simulink model "HybridMicrogrid_FuzzyLogic"  (R2024b)
settings: Solver=ode23tb  StartTime=0.0  StopTime=86000  RelTol=1e-3
PreLoadFcn:
  | addpath('Resources')
InitFcn:
  | initialConditions();
libraries: simulink x6, spsThreePhaseDynamicLoadLib x4, spsThreePhaseVIMeasurementLib x4, spsPower3phPhasorLib x3, spsThreePhaseBreakerLib x3, spsThreePhaseSourceLib x2, fuzblock x2, spsFrequencyPhasorLib x2, spsSequenceAnalyzerPhasorLib x2, powerlib_meascontrol x1, powerlib x1, spsCurrentMeasurementLib x1
settings Model: SimulationMode=accelerator  Creator=jlesage  LastModifiedBy=RDBNTO016
settings SolverCC: ZeroCrossAlgorithm=Adaptive  AlgebraicLoopSolver=TrustRegion
settings DataIOCC: ReturnWorkspaceOutputs=off
settings DebuggingCC: IgnoredZcDiagnostic=none  PregeneratedLibrarySubsystemCodeDiagnostic=none  ArithmeticOperatorsInVariantConditions=warning
settings ModelReferenceCC: EnableRefExpFcnMdlSchedulingChecks=on
settings SFSimCC: SimUseLocalCustomCode=off  CustomCodeUndefinedFunction=UseInterfaceOnly
settings RTWCC: RTWUseLocalCustomCode=off  GPUComputeCapability=3.5

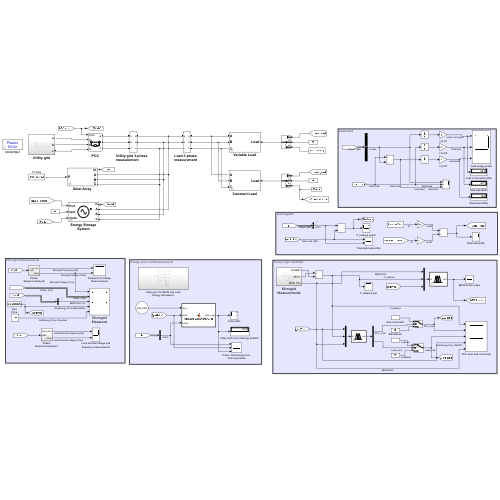
[thumbnail: Simulink's stored preview of the top-level diagram]
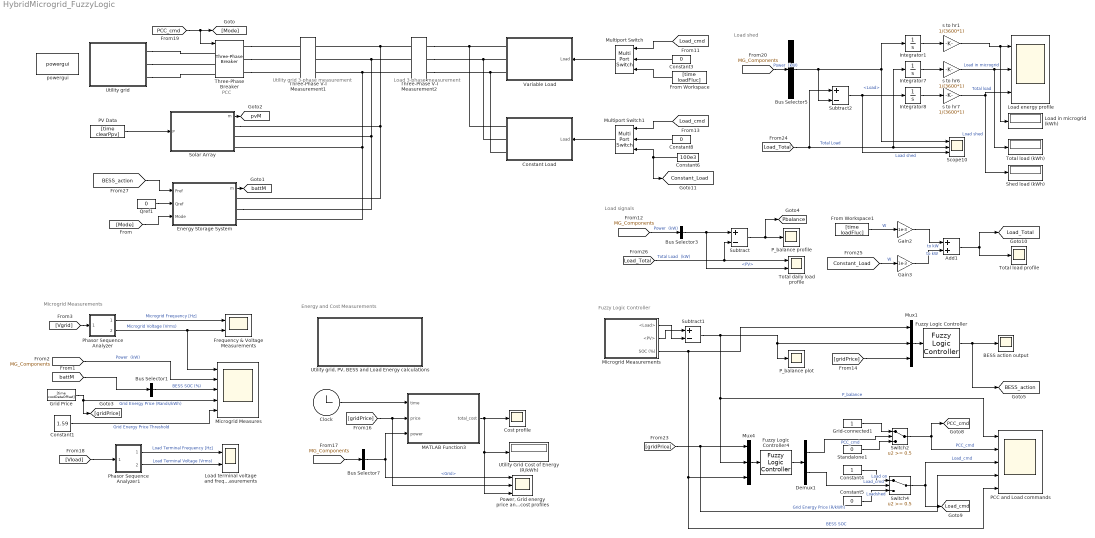
== system HybridMicrogrid_FuzzyLogic ==
  note: PCC
  note: Energy and Cost Measurements
  note: Fuzzy Logic Controller
  note: Microgrid Measurements
  note: Load shed
  note: Load 3-phase measurement
  note: Utility grid 3-phase measurement
  note: Load signals
  Add1 : Sum
  BESS action output : Scope
  Bus Selector1 : BusSelector  OutputSignals=SOC (%)  OutputAsBus=on
  Bus Selector3 : BusSelector  OutputSignals=PV
  Bus Selector5 : BusSelector  OutputSignals=Load
  Bus Selector7 : BusSelector  OutputSignals=Grid
  Clock : Clock
  Constant Load : Subsystem  mask(Variable Load (PQ Model)){Vn=400, Fn=50, PF=1, Load0=0}
      mask prompts: Vn "Nominal L-L Voltage [Vrms]"; Fn "Nominal Frequency [Hz]"; PF "Power Factor [0 to 1]"; Load0 "Initial Load [W]"
      mask help:
      | The Variable Load block is a lumped approximation for a distribution feeder. For non-unity power factor loads, the input (active power) is scaled accordingly to generate a desired load.
      |
      | Note: The initial input load must be specified for use for Load Flow analysis.
      mask init:
      | P0 = Load0;
      | Q0 = Load0*sqrt(1/PF^2-1);
      mask Display:
      | port_label('input',1,'Load')
      | port_label('Rconn',1,'A')
      | port_label('Rconn',2,'B')
      | port_label('Rconn',3,'C')
  Constant1 : Constant  Value=1.59
  Constant3 : Constant  Value=0
  Constant4 : Constant
  Constant5 : Constant  Value=0
  Constant6 : Constant  Value=100e3
  Constant8 : Constant  Value=0
  Cost profile : Scope
  Demux1 : Demux  Outputs=2
  Energy Storage System : Subsystem  mask(Grid-connected Energy Storage (PQ Model)){SimMode=Phasor, Vn=400, Fn=50, PnomkW=300, kWh_Rated=3000, Efficiency=96, LimitVec=[90 30], RechargeSOC=50, Precharge=90, autoRecharge=on, Initial_kWh_pc=50, PQvec=[300e3 0]}
      mask prompts: SimMode "Simulation Mode"; Vn "Nominal L-L Voltage [Vrms]"; Fn "Nominal Frequency [Hz]"; PnomkW "Rated Power [kW]"; kWh_Rated "Rated Capacity [kWh]"; Efficiency "Overall System Efficiency [%]"; LimitVec "Upper/Lower Charge Limits [%]"; RechargeSOC "SOC to Recharge [%]"; Precharge "Recharge Rate [% of Rated Power]"; autoRecharge "Enable Auto-Recharge"; Initial_kWh_pc "Initial State-of-Charge [0-100%]"; PQvec "Initial Active/Reactive Cmds"
      mask help:
      | The energy storage block models a generic grid-connected energy storage system (ESS), most commonly a battery system. This is a system-level model that does not contain any power electronics, but is useful for load flow, phasor, and hybrid phasor-EMT simulations. The inputs to this block are the commanded active and reactive power of the ESS. The ESS is assumed to have four quadrent operation. The Mode Input dictates what high-level operation the ESS has: current control (Mode = 1) or voltage control (Mode = 0). Current control is ideal for a grid connected system where you need to specify P,Q commands. Voltage control is necessary if the ESS will be the only system supporting the microgrid in islanded mode.
      |
      | For more detailed ESS models, consider the battery block in the Drives library. Consider using this PQ Model to perform load flow studies and switch to a more detailed model when full EMT studies or more advanced controls are required.
      |
      | Note: The initial active/reactive power commands must be specified for use for Load Flow analysis.
      mask init:
      | % Calculate Initial Conditions
      | Pnom = PnomkW*1e3;
      | P0 = -PQvec(1);  Q0 = -PQvec(2);
      | if abs(P0) > Pnom
      |     P0 = sign(P0)*Pnom;
      | end
      | 
      | % Calculate Q0 given Reactive Power Capability Curve
      | Qlim = sqrt(Pnom^2 - P0^2);
      | if Qlim > abs(Q0)
      |     Q0 = sign(Q0)*Qlim;
      | end
      | 
      | UpChrgLim = LimitVec(1);
      | LowChrgLim = LimitVec(2);
      | if Initial_kWh_pc > UpChrgLim && P0 < 0
      |     P0 = 0; Q0 = 0;
      | elseif Initial_kWh_pc < LowChrgLim && P0 > 0
      |     P0 = 0; Q0 = 0;
      | end
      | 
      | simulationStatus =  get_param(bdroot,'SimulationStatus');
      | 
      | % The active variant can only be modified at edit-time or very early during
      | % the simulink compile stage. 
      | if any(strcmp(simulationStatus, {'stopped'}))
      | 
      | blk = [gcb '/Power Measures'];
      | if strcmp(SimMode,'Phasor')
      |     set_param(blk,'OverrideUsingVariant','Phasor');
      | else
      |     set_param(blk,'OverrideUsingVariant','EMT');
      | end
      | 
      | 
      | end
      mask TypeOptions SimMode: Electromagnetic Transient (EMT) | Phasor
      mask DialogControl Container7 Prompt: Grid Connection Properties
      mask DialogControl Container11 Prompt: Charge/Discharge Controls
      mask DialogControl Container12 Prompt: Initial Conditions
      mask Display: plot(-80,-50,80,50,[0,9,18,24,29,30,29,24,18,9,0,-9,-18,-24,-29,-30,-29,-24,-18,-9,0],[30,29,24,18,9,0,-9,-18,-24,-29,-30,-29,-24,-18,-9,0,9,18,24,29,30],[-50],[0],[50],[0],[45 35 40 40 40],[15 15 15 20 10],[1 2 3 4 5 6 7 8 9 10 11 12 13 14 15 16 17 18 19 20 21].*1.5-15,[0,9,18,24,29,30,29,24,18,9,0,-9,-18,-24,-29,-30,-29,-24,-18,-9,0]./2.4)
  Frequency & Voltage Measurements : Scope  NumInputPorts=2
  From Workspace : FromWorkspace  VariableName=[time loadFluc]
  From Workspace1 : FromWorkspace  VariableName=[time loadFluc]
  Fuzzy Logic Controller : fuzblock/Fuzzy Logic  Controller  FIS=Fuzzy_EMS  OutputSampleNumber=101  DataType=double  FuzzifiedInputs=off  RuleFiringStrengths=off  RuleOutputs=off  AggregatedOutputs=off  SimulateUsing=Interpreted execution  OutOfRangeInputValueMessage=warning  NoRuleFiredMessage=warning  EmptyOutputFuzzySetMessage=warning
  Fuzzy Logic Controller4 : fuzblock/Fuzzy Logic  Controller  FIS=Fuzzy_PCC_Load  OutputSampleNumber=101  DataType=double  FuzzifiedInputs=off  RuleFiringStrengths=off  RuleOutputs=off  AggregatedOutputs=off  SimulateUsing=Interpreted execution  OutOfRangeInputValueMessage=warning  NoRuleFiredMessage=warning  EmptyOutputFuzzySetMessage=warning
  Gain2 : Gain  Gain=1e-3
  Gain3 : Gain  Gain=1e-3
  Grid Price : FromWorkspace  VariableName=[time costDataOffset]
  Grid-connected1 : Constant
  Integrator1 : Integrator
  Integrator7 : Integrator
  Integrator8 : Integrator
  Load energy profile : Scope  NumInputPorts=3
  Load in microgrid (kWh) : Display
  Load terminal voltage and frequency measurements : Scope  NumInputPorts=2
  MATLAB Function3 : MATLAB Function  TreatAsAtomicUnit=on
  Microgrid Measurements : Subsystem
  Microgrid Measures : Scope  NumInputPorts=5
  Multiport Switch : MultiPortSwitch  DataPortOrder=Zero-based contiguous  Inputs=2  zeroidx=on  SaturateOnIntegerOverflow=off  InputSameDT=off
  Multiport Switch1 : MultiPortSwitch  DataPortOrder=Zero-based contiguous  Inputs=2  zeroidx=on  SaturateOnIntegerOverflow=off  InputSameDT=off
  Mux1 : Mux  Inputs=3
  Mux4 : Mux  Inputs=3
  PCC and Load commands : Scope  NumInputPorts=5
  PV Data : FromWorkspace  VariableName=[time clearPpv]
  P_balance plot : Scope
  P_balance profile : Scope
  Phasor Sequence Analyzer : Subsystem
  Phasor Sequence Analyzer1 : Subsystem
  "Power, Grid energy price and cost profiles" : Scope  NumInputPorts=3
  Qref1 : Constant  Value=0
  Scope10 : Scope  NumInputPorts=3
  Shed load (kWh) : Display
  Solar Array : Subsystem  mask(Grid-Connected PV Array (PQ Model)){Vn=400, Fn=50, P0=250e3}
      mask prompts: Vn "Nominal L-L Voltage [Vrms]"; Fn "Nominal Frequency [Hz]"; P0 "Initial Power [W]"
      mask help:
      | This block models a grid-connected solar array using the Three-Phase Dynamic Load block. This is a system-level model that does not contain any power electronics, but is useful for load flow, phasor, and hybrid phasor-EMT simulations. The input to this block is the power output of the grid connected PV array, not irradiance.
      |
      | For more detailed PV models, consider the PV Array block in the Renewables library. Consider using this PQ Model to perform load flow studies and switch to a more detailed model when full EMT studies are required.
      |
      | Note: The array power must be specified for use for Load Flow analysis.
      mask init:
      | % P0 = Irr0*TotalArea*Efficiency/100;
      | P0 = -P0;
      mask Display:
      | port_label('input',1,'P')
      | port_label('output',1,'m')
      | port_label('Rconn',1,'A')
      | port_label('Rconn',2,'B')
      | port_label('Rconn',3,'C')
  Standalone1 : Constant  Value=0
  Subtract : Sum  Inputs=+-
  Subtract1 : Sum  Inputs=+-
  Subtract2 : Sum  Inputs=+-
  Switch2 : Switch  Threshold=0.5  SaturateOnIntegerOverflow=off  InputSameDT=off
  Switch4 : Switch  Threshold=0.5  SaturateOnIntegerOverflow=off  InputSameDT=off
  Three-Phase V-I Measurement1 : spsThreePhaseVIMeasurementLib/Three-Phase V-I Measurement  VoltageMeasurement=phase-to-ground  SetLabelV=on  LabelV=Vgrid  Vpu=off  VpuLL=off  CurrentMeasurement=yes  SetLabelI=on  LabelI=Igrid  Ipu=off  Pbase=100e6  Vbase=500e3  OutputType=Complex  PhasorSimulation=on  PSBequivalent=0
  Three-Phase V-I Measurement2 : spsThreePhaseVIMeasurementLib/Three-Phase V-I Measurement  VoltageMeasurement=phase-to-ground  SetLabelV=on  LabelV=Vload  Vpu=off  VpuLL=off  CurrentMeasurement=yes  SetLabelI=on  LabelI=Iload  Ipu=off  Pbase=100e6  Vbase=500e3  OutputType=Complex  PhasorSimulation=on  PSBequivalent=0
  Three-Phase Breaker : spsThreePhaseBreakerLib/Three-Phase Breaker  InitialState=closed  SwitchA=on  SwitchB=on  SwitchC=on  SwitchTimes="[1/60  5/60]"  External=on  BreakerResistance=0.01  SnubberResistance=1e6  SnubberCapacitance=inf  Measurements=None
  Total daily load profile : Scope  NumInputPorts=2
  Total load (kWh) : Display
  Total load profile : Scope
  Utility Grid Cost of Energy (R/kWh) : Display
  Utility grid : Subsystem
  "Utility grid, PV, BESS and Load Energy calculations" : Subsystem
  Variable Load : Subsystem  mask(Variable Load (PQ Model)){Vn=400, Fn=50, PF=1, Load0=0}
      mask prompts: Vn "Nominal L-L Voltage [Vrms]"; Fn "Nominal Frequency [Hz]"; PF "Power Factor [0 to 1]"; Load0 "Initial Load [W]"
      mask help:
      | The Variable Load block is a lumped approximation for a distribution feeder. For non-unity power factor loads, the input (active power) is scaled accordingly to generate a desired load.
      |
      | Note: The initial input load must be specified for use for Load Flow analysis.
      mask init:
      | P0 = Load0;
      | Q0 = Load0*sqrt(1/PF^2-1);
      mask Display:
      | port_label('input',1,'Load')
      | port_label('Rconn',1,'A')
      | port_label('Rconn',2,'B')
      | port_label('Rconn',3,'C')
  powergui : sps_lib/powergui  Priority=1  SimulationMode=Phasor  SampleTime=1e-4  frequency=50  Iterations=50  frequencyindice=50  Pbase=100e6  ErrMax=0.0001  UnitsV=kV  UnitsW=MW  buscounter=3  FunctionMessages=off  echomessages=off  EnableUseOfTLC=off  CurrentSourceSwitches=off  DisableSnubberDevices=off  DisableRonSwitches=off  DisableVfSwitches=off  DisplayEquations=off  AutomaticDiscreteSolvers=off  SolverType=Tustin/Backward Euler (TBE)  Interpol=off  ExternalGateDelay=off  methode=off  Ts=100  x0status=blocks  SPID=on  SwTol=0  HookPort=off  NonlinearTolerance=0  nMaxIteration=15  ContinueOnMaxIteration=off  RestoreLinks=warning  ResistiveCurrentMeasurement=off  Frange=[0:2:500]  Ylog=off  Xlog=on  ShowGrid=off  save=off  variable=ZData  structure=0  ZoomFFT=off  StartTime=0.0  cycles=1  DisplayStyle=1  fundamental=60  FreqAxis=off  MaxFrequency=1000  frequencyindicesteady=1  RmsSteady=1  display=off
  s to hr1 : Gain  Gain=1/(3600*1)
  s to hr6 : Gain  Gain=1/(3600*1)
  s to hr7 : Gain  Gain=1/(3600*1)
  tag scope: BESS_action=global, Constant_Load=global, Load_Total=global, Load_cmd=global, PCC_cmd=global, Pbalance=global, battM=global, pvM=global
  wires:
  Qref1/1 -> Energy Storage System/2(Qref)
  Energy Storage System/1(m) -> [battM]
  Solar Array/1(m) -> [pvM]
  [Vgrid] -> Phasor Sequence Analyzer/1(Vabc)
  [Mode] -> Energy Storage System/3(Mode)
  [MG_Components] -> Microgrid Measures/2  "Power  (kW)"
  Phasor Sequence Analyzer/2(Vrms) -> Microgrid Measures/1, Frequency & Voltage Measurements/2  "Microgrid Voltage (Vrms)"
  [battM] -> Bus Selector1/1
  Bus Selector1/1 -> Microgrid Measures/3  "BESS SOC (%)"
  Phasor Sequence Analyzer/1(Freq (Hz)) -> Frequency & Voltage Measurements/1  "Microgrid Frequency [Hz]"
  Grid Price/1 -> [gridPrice], Microgrid Measures/4  "Grid Energy Price (Rands/kWh)"
  Fuzzy Logic Controller/1 -> [BESS_action], BESS action output/1
  Subtract/1 -> [Pbalance], P_balance profile/1
  Bus Selector3/1 -> Total daily load profile/2, Subtract/1  "<PV>"
  Microgrid Measurements/1(<Load>) -> Subtract1/2
  Mux1/1 -> Fuzzy Logic Controller/1
  Microgrid Measurements/3(SOC (%)) -> Mux1/1, Mux4/3, PCC and Load commands/5  "BESS SOC"
  Microgrid Measurements/2(<PV>) -> Subtract1/1
  Subtract1/1 -> Mux4/2, PCC and Load commands/1, Mux1/2, P_balance plot/1  "P_balance"
  Constant1/1 -> Microgrid Measures/5  "Grid Energy Price Threshold"
  Clock/1 -> MATLAB Function3/1(time)
  [gridPrice] -> "Power, Grid energy price and cost profiles"/2, MATLAB Function3/2(price)
  [MG_Components] -> Bus Selector7/1
  Bus Selector7/1 -> "Power, Grid energy price and cost profiles"/1, MATLAB Function3/3(power)  "<Grid>"
  MATLAB Function3/1(total_cost) -> Cost profile/1, Utility Grid Cost of Energy (R/kWh)/1, "Power, Grid energy price and cost profiles"/3
  PV Data/1 -> Solar Array/1(P)
  [MG_Components] -> Bus Selector3/1  "Power  (kW)"
  Multiport Switch/1 -> Variable Load/1(Load)
  Constant3/1 -> Multiport Switch/2
  [Load_cmd] -> Multiport Switch/1
  Mux4/1 -> Fuzzy Logic Controller4/1
  [gridPrice] -> PCC and Load commands/4, Mux4/1  "Grid Energy Price (R/kWh)"
  Fuzzy Logic Controller4/1 -> Demux1/1
  Demux1/1 -> Switch2/2  "PCC_cmd"
  Demux1/2 -> Switch4/2  "Load_cmd"
  Constant5/1 -> Switch4/3  "Loadshed"
  Constant4/1 -> Switch4/1  "Load on"
  Switch4/1 -> [Load_cmd], PCC and Load commands/3  "Load_cmd"
  Grid-connected1/1 -> Switch2/1
  Standalone1/1 -> Switch2/3
  From Workspace/1 -> Multiport Switch/3
  [MG_Components] -> Bus Selector5/1  "Power  (kW)"
  Bus Selector5/1 -> Integrator1/1, Scope10/1, Subtract2/2  "<Load>"
  [Load_Total] -> Subtract2/1, Integrator7/1, Scope10/2  "Total Load"
  Subtract2/1 -> Scope10/3, Integrator8/1  "Load shed"
  Integrator1/1 -> s to hr1/1
  s to hr1/1 -> Load in microgrid (kWh)/1, Load energy profile/1  "Load in microgrid"
  Integrator8/1 -> s to hr7/1
  s to hr7/1 -> Shed load (kWh)/1, Load energy profile/3  "Load shed"
  Integrator7/1 -> s to hr6/1
  s to hr6/1 -> Total load (kWh)/1, Load energy profile/2  "Total load"
  [Load_cmd] -> Multiport Switch1/1
  Multiport Switch1/1 -> Constant Load/1(Load)
  Constant8/1 -> Multiport Switch1/2
  Constant6/1 -> [Constant_Load], Multiport Switch1/3
  [Constant_Load] -> Gain3/1  "W"
  From Workspace1/1 -> Gain2/1  "W"
  Gain2/1 -> Add1/1  "to kW"
  Gain3/1 -> Add1/2  "to kW"
  Add1/1 -> Total load profile/1, [Load_Total]
  [Load_Total] -> Total daily load profile/1, Subtract/2  "Total Load  (kW)"
  [PCC_cmd] -> Three-Phase Breaker/1, [Mode]
  [gridPrice] -> Mux1/3
  [BESS_action] -> Energy Storage System/1(Pref)
  [Vload] -> Phasor Sequence Analyzer1/1(Vabc)
  Phasor Sequence Analyzer1/1(Freq (Hz)) -> Load terminal voltage and frequency measurements/1  "Load Terminal Frequency [Hz]"
  Phasor Sequence Analyzer1/2(Vrms) -> Load terminal voltage and frequency measurements/2  "Load Terminal Voltage (Vrms)"
  Switch2/1 -> [PCC_cmd], PCC and Load commands/2  "PCC_cmd"
  connections:
  Variable Load/RConn2 -- Three-Phase V-I Measurement2/LConn2 -- Constant Load/RConn2
  Solar Array/RConn3 -- Energy Storage System/RConn3 -- Three-Phase V-I Measurement2/RConn3 -- Three-Phase V-I Measurement1/RConn3
  Three-Phase Breaker/RConn1 -- Three-Phase V-I Measurement1/LConn1
  Three-Phase Breaker/RConn2 -- Three-Phase V-I Measurement1/LConn2
  Three-Phase Breaker/RConn3 -- Three-Phase V-I Measurement1/LConn3
  Variable Load/RConn1 -- Three-Phase V-I Measurement2/LConn1 -- Constant Load/RConn1
  Solar Array/RConn1 -- Energy Storage System/RConn1 -- Three-Phase V-I Measurement2/RConn1 -- Three-Phase V-I Measurement1/RConn1
  Energy Storage System/RConn2 -- Three-Phase V-I Measurement2/RConn2 -- Three-Phase V-I Measurement1/RConn2 -- Solar Array/RConn2
  Variable Load/RConn3 -- Three-Phase V-I Measurement2/LConn3 -- Constant Load/RConn3
  Utility grid/RConn1 -- Three-Phase Breaker/LConn1
  Utility grid/RConn2 -- Three-Phase Breaker/LConn2
  Utility grid/RConn3 -- Three-Phase Breaker/LConn3

== system HybridMicrogrid_FuzzyLogic/Constant Load ==
  Load : Inport
  Dynamic Load Control : Subsystem
  Simple Three-Phase Load : spsThreePhaseDynamicLoadLib/Three-Phase Dynamic Load  NominalVoltage=[Vn Fn]  ActiveReactivePowers=[200000 45883.1]  PositiveSequence=[0.999844 -0.0038635]  ExternalControl=on  NpNq=[1.3 2]  TimeConstants="[0  0  0  0]"  MinimumVoltage=0.7  Tfilter=1e-2  LoadFlowParameters=[4,0,0,0,0]
  Terminator : Terminator
  A : PMIOPort  Side=Right
  B : PMIOPort  Port=2  Side=Right
  C : PMIOPort  Port=3  Side=Right
  wires:
  Dynamic Load Control/1(PQ) -> Simple Three-Phase Load/1
  Load/1 -> Dynamic Load Control/1(P0)
  Simple Three-Phase Load/1 -> Terminator/1
  connections:
  Simple Three-Phase Load/LConn2 -- B/RConn1
  Simple Three-Phase Load/LConn3 -- C/RConn1
  Simple Three-Phase Load/LConn1 -- A/RConn1

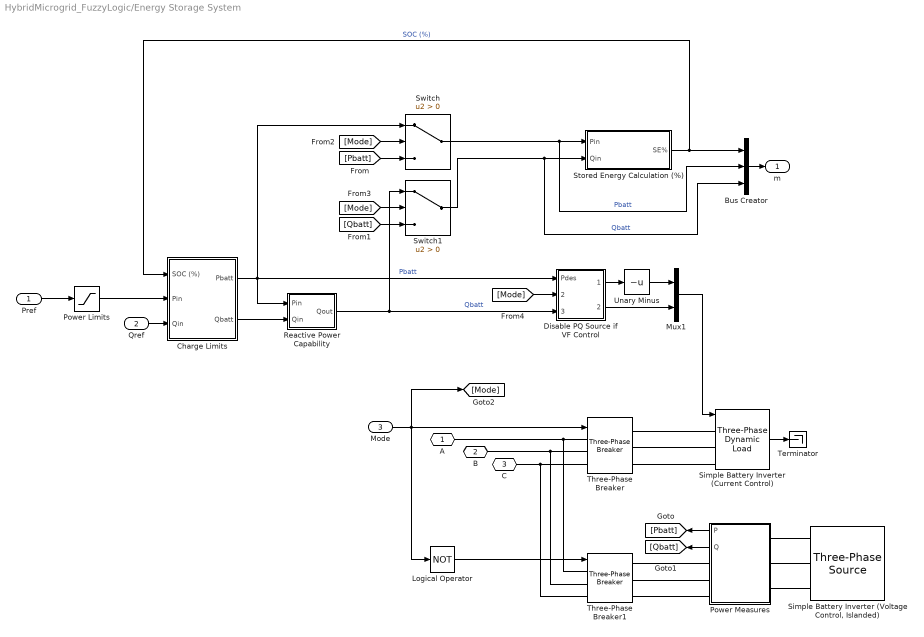
== system HybridMicrogrid_FuzzyLogic/Energy Storage System ==
  Pref : Inport
  Qref : Inport  Port=2
  Mode : Inport  Port=3
  Bus Creator : BusCreator  Inputs=3
  Charge Limits : Subsystem
  Disable PQ Source if VF Control : Subsystem
  Logical Operator : Logic  Operator=NOT  AllPortsSameDT=off  OutDataTypeStr=boolean
  Mux1 : Mux  Inputs=2
  Power Limits : Saturate  UpperLimit=Pnom  LowerLimit=-Pnom
  Power Measures : Subsystem  Variant=on  VariantControlMode=label  LabelModeActiveChoice=Phasor
  Reactive Power Capability : Subsystem
  Simple Battery Inverter (Current Control) : spsThreePhaseDynamicLoadLib/Three-Phase Dynamic Load  NominalVoltage=[Vn Fn]  ActiveReactivePowers=[-100e3 -3.38813e-13]  PositiveSequence=[0.999844 -0.0038635]  ExternalControl=on  NpNq=[1.3 2]  TimeConstants="[0  0  0  0]"  MinimumVoltage=0.7  Tfilter=1e-2  LoadFlowParameters=[4,0,0,0,0]
      settings: LibrarySourceBlock=|
      | sps_lib/Passives/Three-Phase
      | Dynamic Load
  "Simple Battery Inverter (Voltage Control, Islanded)" : spsThreePhaseSourceLib/Three-Phase Source  InternalConnection=Yg  VoltagePhases=off  Voltage=Vn  PhaseAngle=0  Voltage_phases=[25e3 25e3 25e3]/sqrt(3)  PhaseAngles_phases=[0 -120 +120]  Frequency=Fn  NonIdealSource=off  SpecifyImpedance=off  Resistance=0.8929  Inductance=16.58e-3  ShortCircuitLevel=100e6  BaseVoltage=25e3  XRratio=7  BusType=swing  Pref=10e3  Qref=0  Prefabc=[10e3, 10e3, 10e3]  Qrefabc=[0, 0, 0]  Qmin=-inf  Qmax=inf
  Stored Energy Calculation (%) : Subsystem
  Switch : Switch  Criteria=u2 > Threshold  SaturateOnIntegerOverflow=off  InputSameDT=off
  Switch1 : Switch  Criteria=u2 > Threshold  SaturateOnIntegerOverflow=off  InputSameDT=off
  Terminator : Terminator
  Three-Phase Breaker : spsThreePhaseBreakerLib/Three-Phase Breaker  InitialState=closed  SwitchA=on  SwitchB=on  SwitchC=on  SwitchTimes="[1/60  5/60]"  External=on  BreakerResistance=0.01  SnubberResistance=1e6  SnubberCapacitance=inf  Measurements=None
  Three-Phase Breaker1 : spsThreePhaseBreakerLib/Three-Phase Breaker  InitialState=open  SwitchA=on  SwitchB=on  SwitchC=on  SwitchTimes="[1/60  5/60]"  External=on  BreakerResistance=0.01  SnubberResistance=1e6  SnubberCapacitance=inf  Measurements=None
  Unary Minus : UnaryMinus
  A : PMIOPort  Side=Right
  B : PMIOPort  Port=2  Side=Right
  C : PMIOPort  Port=3  Side=Right
  m : Outport  VectorParamsAs1DForOutWhenUnconnected=off
  wires:
  Charge Limits/2(Qbatt) -> Reactive Power Capability/2(Qin)
  Qref/1 -> Charge Limits/3(Qin)
  Power Limits/1 -> Charge Limits/2(Pin)
  Stored Energy Calculation (%)/1(SE%) -> Bus Creator/1, Charge Limits/1(SOC (%))  "SOC (%)"
  Bus Creator/1 -> m/1
  Pref/1 -> Power Limits/1
  Simple Battery Inverter (Current Control)/1 -> Terminator/1
  Mux1/1 -> Simple Battery Inverter (Current Control)/1
  Unary Minus/1 -> Mux1/1
  Logical Operator/1 -> Three-Phase Breaker1/1
  Mode/1 -> [Mode], Logical Operator/1, Three-Phase Breaker/1
  Power Measures/1(P) -> [Pbatt]
  Power Measures/2(Q) -> [Qbatt]
  Switch/1 -> Bus Creator/2, Stored Energy Calculation (%)/1(Pin)  "Pbatt"
  Switch1/1 -> Bus Creator/3, Stored Energy Calculation (%)/2(Qin)  "Qbatt"
  [Mode] -> Switch/2
  [Mode] -> Switch1/2
  [Qbatt] -> Switch1/3
  [Pbatt] -> Switch/3
  Charge Limits/1(Pbatt) -> Switch/1, Reactive Power Capability/1(Pin), Disable PQ Source if VF Control/1(Pdes)  "Pbatt"
  [Mode] -> Disable PQ Source if VF Control/2(Mode)
  Reactive Power Capability/1(Qout) -> Disable PQ Source if VF Control/3(Qdes), Switch1/1  "Qbatt"
  Disable PQ Source if VF Control/1(Pbatt) -> Unary Minus/1
  Disable PQ Source if VF Control/2(Qbatt) -> Mux1/2
  connections:
  Three-Phase Breaker/RConn1 -- Simple Battery Inverter (Current Control)/LConn1
  Three-Phase Breaker/RConn2 -- Simple Battery Inverter (Current Control)/LConn2
  Three-Phase Breaker/RConn3 -- Simple Battery Inverter (Current Control)/LConn3
  Three-Phase Breaker/LConn3 -- Three-Phase Breaker1/LConn3 -- C/RConn1
  Three-Phase Breaker/LConn2 -- B/RConn1 -- Three-Phase Breaker1/LConn2
  Three-Phase Breaker/LConn1 -- A/RConn1 -- Three-Phase Breaker1/LConn1
  Power Measures/LConn1 -- "Simple Battery Inverter (Voltage Control, Islanded)"/RConn1
  Power Measures/RConn1 -- Three-Phase Breaker1/RConn1
  Power Measures/LConn2 -- "Simple Battery Inverter (Voltage Control, Islanded)"/RConn2
  Power Measures/RConn2 -- Three-Phase Breaker1/RConn2
  Power Measures/LConn3 -- "Simple Battery Inverter (Voltage Control, Islanded)"/RConn3
  Power Measures/RConn3 -- Three-Phase Breaker1/RConn3

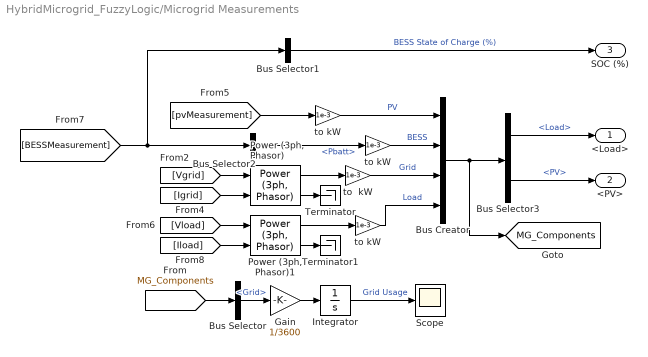
== system HybridMicrogrid_FuzzyLogic/Microgrid Measurements ==
  " to kW" : Gain  Gain=1e-3
  Bus Creator : BusCreator  Inputs=4
  Bus Selector : BusSelector  OutputSignals=Grid
  Bus Selector1 : BusSelector  OutputSignals=SOC (%)  OutputAsBus=on
  Bus Selector2 : BusSelector  OutputSignals=Pbatt
  Bus Selector3 : BusSelector  OutputSignals=Load,PV
  Gain : Gain  Gain=1/3600
  Integrator : Integrator
  "Power (3ph, Phasor)" : spsPower3phPhasorLib/Power (3ph, Phasor)
      settings: LibrarySourceBlock=|
      | sps_lib/Sensors and Measurements/Power
      | (3ph, Phasor)
  "Power (3ph, Phasor)1" : spsPower3phPhasorLib/Power (3ph, Phasor)
      settings: LibrarySourceBlock=|
      | sps_lib/Sensors and Measurements/Power
      | (3ph, Phasor)
  Scope : Scope
  Terminator : Terminator
  Terminator1 : Terminator
  to  kW : Gain  Gain=1e-3
  to kW : Gain  Gain=1e-3
  "to kW " : Gain  Gain=1e-3
  <Load> : Outport  VectorParamsAs1DForOutWhenUnconnected=off
  <PV> : Outport  Port=2  VectorParamsAs1DForOutWhenUnconnected=off
  SOC (%) : Outport  Port=3  VectorParamsAs1DForOutWhenUnconnected=off
  tag scope: MG_Components=global
  wires:
  Bus Creator/1 -> [MG_Components], Bus Selector3/1
  "Power (3ph, Phasor)1"/2 -> Terminator1/1
  " to kW"/1 -> Bus Creator/4  "Load"
  "to kW "/1 -> Bus Creator/2  "BESS"
  [Vload] -> "Power (3ph, Phasor)1"/1
  "Power (3ph, Phasor)"/2 -> Terminator/1
  [pvMeasurement] -> to kW/1
  [Iload] -> "Power (3ph, Phasor)1"/2
  [Igrid] -> "Power (3ph, Phasor)"/2
  Bus Selector2/1 -> "to kW "/1  "<Pbatt>"
  [Vgrid] -> "Power (3ph, Phasor)"/1
  to kW/1 -> Bus Creator/1  "PV"
  "Power (3ph, Phasor)"/1 -> to  kW/1
  "Power (3ph, Phasor)1"/1 -> " to kW"/1
  to  kW/1 -> Bus Creator/3  "Grid"
  Bus Selector1/1 -> SOC (%)/1  "BESS State of Charge (%)"
  Bus Selector3/2 -> <PV>/1  "<PV>"
  Bus Selector3/1 -> <Load>/1  "<Load>"
  [BESSMeasurement] -> Bus Selector1/1, Bus Selector2/1
  [MG_Components] -> Bus Selector/1
  Bus Selector/1 -> Gain/1  "<Grid>"
  Integrator/1 -> Scope/1  "Grid Usage"
  Gain/1 -> Integrator/1

== system HybridMicrogrid_FuzzyLogic/Phasor Sequence Analyzer ==
  Vabc : Inport
  Frequency (Phasor) : spsFrequencyPhasorLib/Frequency (Phasor)  Fn=50  T=0.1
      settings: LibrarySourceBlock=|
      | sps_lib/Sensors and Measurements/Frequency
      | (Phasor)
  LG to LL : Gain  Gain=sqrt(3)/sqrt(2)
  Sequence Analyzer (Phasor) : spsSequenceAnalyzerPhasorLib/Sequence Analyzer (Phasor)  seq=Positive
      settings: LibrarySourceBlock=|
      | sps_lib/Sensors and Measurements/Sequence Analyzer
      | (Phasor)
  Terminator : Terminator
  deg-to-rad : Gain  Gain=pi/180
  Freq (Hz) : Outport  VectorParamsAs1DForOutWhenUnconnected=off
  Vrms : Outport  Port=2  VectorParamsAs1DForOutWhenUnconnected=off
  wires:
  Sequence Analyzer (Phasor)/1 -> LG to LL/1
  Vabc/1 -> Sequence Analyzer (Phasor)/1
  Sequence Analyzer (Phasor)/2 -> deg-to-rad/1
  deg-to-rad/1 -> Frequency (Phasor)/1
  Frequency (Phasor)/1 -> Freq (Hz)/1
  Frequency (Phasor)/2 -> Terminator/1
  LG to LL/1 -> Vrms/1

== system HybridMicrogrid_FuzzyLogic/Phasor Sequence Analyzer1 ==
  Vabc : Inport
  Frequency (Phasor) : spsFrequencyPhasorLib/Frequency (Phasor)  Fn=50  T=0.1
  LG to LL : Gain  Gain=sqrt(3)/sqrt(2)
  Sequence Analyzer (Phasor) : spsSequenceAnalyzerPhasorLib/Sequence Analyzer (Phasor)  seq=Positive
  Terminator : Terminator
  deg-to-rad : Gain  Gain=pi/180
  Freq (Hz) : Outport  VectorParamsAs1DForOutWhenUnconnected=off
  Vrms : Outport  Port=2  VectorParamsAs1DForOutWhenUnconnected=off
  wires:
  Sequence Analyzer (Phasor)/1 -> LG to LL/1
  Vabc/1 -> Sequence Analyzer (Phasor)/1
  Sequence Analyzer (Phasor)/2 -> deg-to-rad/1
  deg-to-rad/1 -> Frequency (Phasor)/1
  Frequency (Phasor)/1 -> Freq (Hz)/1
  Frequency (Phasor)/2 -> Terminator/1
  LG to LL/1 -> Vrms/1

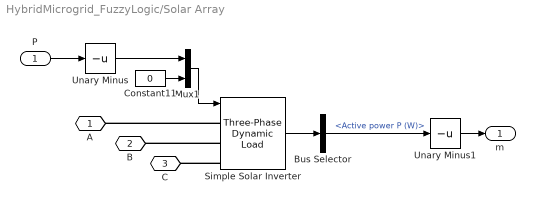
== system HybridMicrogrid_FuzzyLogic/Solar Array ==
  P : Inport
  Bus Selector : BusSelector  OutputSignals=Active power P (W)
  Constant11 : Constant  Value=0
  Mux1 : Mux  Inputs=2
  Simple Solar Inverter : spsThreePhaseDynamicLoadLib/Three-Phase Dynamic Load  NominalVoltage=[Vn Fn]  ActiveReactivePowers=[-250000 -3.38813e-13]  PositiveSequence=[0.999844 -0.0038635]  ExternalControl=on  NpNq=[1.3 2]  TimeConstants="[0  0  0  0]"  MinimumVoltage=0.7  Tfilter=1e-2  LoadFlowParameters=[4,0,0,0,0]
      settings: LibrarySourceBlock=|
      | sps_lib/Passives/Three-Phase
      | Dynamic Load
  Unary Minus : UnaryMinus
  Unary Minus1 : UnaryMinus
  A : PMIOPort  Side=Right
  B : PMIOPort  Port=2  Side=Right
  C : PMIOPort  Port=3  Side=Right
  m : Outport  VectorParamsAs1DForOutWhenUnconnected=off
  wires:
  P/1 -> Unary Minus/1
  Unary Minus/1 -> Mux1/1
  Mux1/1 -> Simple Solar Inverter/1
  Constant11/1 -> Mux1/2
  Simple Solar Inverter/1 -> Bus Selector/1
  Bus Selector/1 -> Unary Minus1/1  "<Active power P (W)>"
  Unary Minus1/1 -> m/1
  connections:
  Simple Solar Inverter/LConn2 -- B/RConn1
  Simple Solar Inverter/LConn3 -- C/RConn1
  Simple Solar Inverter/LConn1 -- A/RConn1

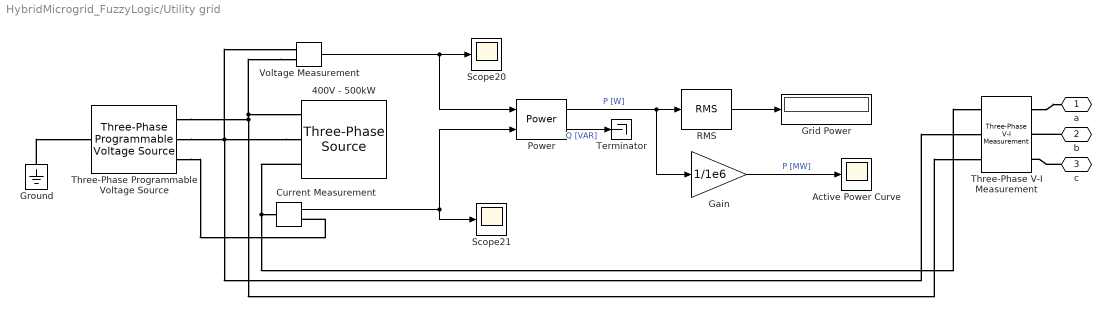
== system HybridMicrogrid_FuzzyLogic/Utility grid ==
  400V - 500kW : spsThreePhaseSourceLib/Three-Phase Source  InternalConnection=Yg  VoltagePhases=off  Voltage=400  PhaseAngle=0  Voltage_phases=[25e3 25e3 25e3]/sqrt(3)  PhaseAngles_phases=[0 -120 +120]  Frequency=50  NonIdealSource=on  SpecifyImpedance=on  Resistance=0.8929  Inductance=16.58e-3  ShortCircuitLevel=500e3  BaseVoltage=400  XRratio=7  BusType=swing  Pref=10e3  Qref=0  Prefabc=[10e3, 10e3, 10e3]  Qrefabc=[0, 0, 0]  Qmin=-inf  Qmax=inf
  Active Power Curve : Scope
  Current Measurement : spsCurrentMeasurementLib/Current Measurement  PhasorSimulation=on  OutputType=Complex  PSBequivalent=0
  Gain : Gain  Gain=1/1e6
  Grid Power : Display
  Ground : spsGroundLib/Ground  LConnTagsString=a
  Power : spsPowerLib/Power  Freq=50  Vinit=[1, 0]  Iinit=[1, 0]  Ts=0
  RMS : spsRMSLib/RMS  TrueRMS=on  Freq=50  RMSInit=120  Ts=0
  Scope20 : Scope
  Scope21 : Scope
  Terminator : Terminator
  Three-Phase Programmable Voltage Source : spsThreePhaseProgrammableVoltageSourceLib/Three-Phase Programmable Voltage Source  PositiveSequence="[440  0 50]"  VariationEntity=None  VariationType=Table of time-amplitude pairs  VariationTypeAlt=Step  VariationStep=0.5  VariationRate=10  VariationMagnitude=0.3  VariationFrequency=2  VariationTiming=[1 2]  VariationPhaseA=off  Amplitudes=[1 0.8 1.2 1.0]  TimeValues=[0 0.1 0.15 0.2]  HarmonicGeneration=off  HarmonicA=[3 0.2 -25 0]  HarmonicB=[2 0.15 35 2]  Timing="[0.05  3]"  BusType=swing  Pref=0  Qref=0  Qmin=-inf  Qmax=inf
  Three-Phase V-I Measurement : spsThreePhaseVIMeasurementLib/Three-Phase V-I Measurement  VoltageMeasurement=phase-to-ground  SetLabelV=on  LabelV=Vabc  Vpu=off  VpuLL=off  CurrentMeasurement=yes  SetLabelI=on  LabelI=Iabc  Ipu=off  Pbase=100e6  Vbase=500e3  OutputType=Complex  PhasorSimulation=on  PSBequivalent=0
  Voltage Measurement : spsVoltageMeasurementLib/Voltage Measurement  PhasorSimulation=on  OutputType=Complex  PSBequivalent=0
  a : PMIOPort  Side=Right
  b : PMIOPort  Port=2  Side=Right
  c : PMIOPort  Port=3  Side=Right
  wires:
  Voltage Measurement/1 -> Scope20/1, Power/1
  Current Measurement/1 -> Scope21/1, Power/2
  RMS/1 -> Grid Power/1
  Gain/1 -> Active Power Curve/1  "P [MW]"
  Power/2 -> Terminator/1  "Q [VAR]"
  Power/1 -> Gain/1, RMS/1  "P [W]"
  connections:
  Voltage Measurement/LConn2 -- Three-Phase Programmable Voltage Source/RConn1 -- Three-Phase V-I Measurement/LConn3 -- 400V - 500kW/RConn3
  400V - 500kW/RConn2 -- Three-Phase Programmable Voltage Source/RConn2 -- Voltage Measurement/LConn1 -- Three-Phase V-I Measurement/LConn2
  Current Measurement/LConn1 -- 400V - 500kW/RConn1 -- Three-Phase V-I Measurement/LConn1
  Ground/LConn1 -- Three-Phase Programmable Voltage Source/LConn1
  Three-Phase Programmable Voltage Source/RConn3 -- Current Measurement/RConn1
  c/RConn1 -- Three-Phase V-I Measurement/RConn3
  b/RConn1 -- Three-Phase V-I Measurement/RConn2
  Three-Phase V-I Measurement/RConn1 -- a/RConn1

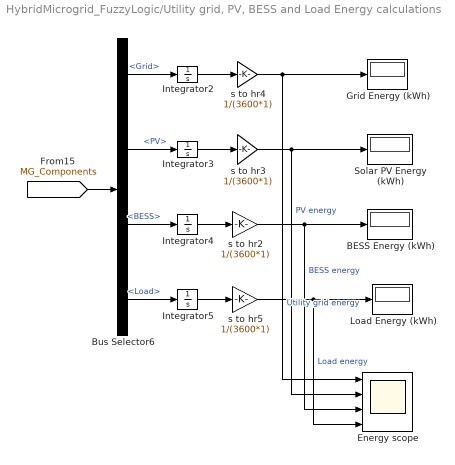
== system HybridMicrogrid_FuzzyLogic/Utility grid, PV, BESS and Load Energy calculations ==
  BESS Energy (kWh) : Display
  Bus Selector6 : BusSelector  OutputSignals=Grid,PV,BESS,Load
  Energy scope : Scope  NumInputPorts=4
  Grid Energy (kWh) : Display
  Integrator{2..5} (4 alike) : Integrator
  Load Energy (kWh) : Display
  Solar PV Energy (kWh) : Display
  s to hr{2..5} (4 alike) : Gain  Gain=1/(3600*1)
  wires:
  Bus Selector6/2 -> Integrator3/1  "<PV>"
  Bus Selector6/3 -> Integrator4/1  "<BESS>"
  Integrator2/1 -> s to hr4/1
  s to hr4/1 -> Grid Energy (kWh)/1, Energy scope/1  "Utility grid energy"
  s to hr2/1 -> BESS Energy (kWh)/1, Energy scope/3  "BESS energy"
  Integrator5/1 -> s to hr5/1
  [MG_Components] -> Bus Selector6/1
  Bus Selector6/1 -> Integrator2/1  "<Grid>"
  Integrator3/1 -> s to hr3/1
  s to hr5/1 -> Load Energy (kWh)/1, Energy scope/4  "Load energy"
  Integrator4/1 -> s to hr2/1
  Bus Selector6/4 -> Integrator5/1  "<Load>"
  s to hr3/1 -> Solar PV Energy (kWh)/1, Energy scope/2  "PV energy"

== system HybridMicrogrid_FuzzyLogic/Variable Load ==
  Load : Inport
  Dynamic Load Control : Subsystem
  Simple Three-Phase Load : spsThreePhaseDynamicLoadLib/Three-Phase Dynamic Load  NominalVoltage=[Vn Fn]  ActiveReactivePowers=[200000 45883.1]  PositiveSequence=[0.999844 -0.0038635]  ExternalControl=on  NpNq=[1.3 2]  TimeConstants="[0  0  0  0]"  MinimumVoltage=0.7  Tfilter=1e-2  LoadFlowParameters=[4,0,0,0,0]
      settings: LibrarySourceBlock=|
      | sps_lib/Passives/Three-Phase
      | Dynamic Load
  Terminator : Terminator
  A : PMIOPort  Side=Right
  B : PMIOPort  Port=2  Side=Right
  C : PMIOPort  Port=3  Side=Right
  wires:
  Simple Three-Phase Load/1 -> Terminator/1
  Load/1 -> Dynamic Load Control/1(P0)
  Dynamic Load Control/1(PQ) -> Simple Three-Phase Load/1
  connections:
  Simple Three-Phase Load/LConn1 -- A/RConn1
  Simple Three-Phase Load/LConn3 -- C/RConn1
  Simple Three-Phase Load/LConn2 -- B/RConn1

== system HybridMicrogrid_FuzzyLogic/Constant Load/Dynamic Load Control ==
  P0 : Inport
  Fcn : Fcn  Expr=sqrt(1/u(1)^2-1)
  Mux : Mux  Inputs=2
  Product : Product
  Summer1 : Constant  Value=PF
  PQ : Outport  VectorParamsAs1DForOutWhenUnconnected=off
  wires:
  Product/1 -> Mux/2  "Qo"
  Mux/1 -> PQ/1
  P0/1 -> Mux/1, Product/1
  Fcn/1 -> Product/2
  Summer1/1 -> Fcn/1

== system HybridMicrogrid_FuzzyLogic/Energy Storage System/Charge Limits ==
  SOC (%) : Inport
  Pin : Inport  Port=2
  Qin : Inport  Port=3
  Overcharge Check : Subsystem
  Undercharge Check : Subsystem
  Pbatt : Outport  VectorParamsAs1DForOutWhenUnconnected=off
  Qbatt : Outport  Port=2  VectorParamsAs1DForOutWhenUnconnected=off
  wires:
  SOC (%)/1 -> Overcharge Check/1(SOC (%)), Undercharge Check/1(SOC (%))
  Undercharge Check/2(Qout) -> Qbatt/1
  Pin/1 -> Overcharge Check/2(Pin)
  Overcharge Check/1(Pout) -> Undercharge Check/2(Pin)
  Qin/1 -> Overcharge Check/3(Qin)
  Undercharge Check/1(Pout) -> Pbatt/1  "Pbatt"
  Overcharge Check/2(Qout) -> Undercharge Check/3(Qin)

== system HybridMicrogrid_FuzzyLogic/Energy Storage System/Disable PQ Source if VF Control ==
  Pdes : Inport
  Mode : Inport  Port=2
  Qdes : Inport  Port=3
  Constant : Constant  Value=0
  Constant1 : Constant  Value=0
  Switch2 : Switch  Criteria=u2 > Threshold  SaturateOnIntegerOverflow=off  InputSameDT=off
  Switch3 : Switch  Criteria=u2 > Threshold  SaturateOnIntegerOverflow=off  InputSameDT=off
  Pbatt : Outport  VectorParamsAs1DForOutWhenUnconnected=off
  Qbatt : Outport  Port=2  VectorParamsAs1DForOutWhenUnconnected=off
  wires:
  Mode/1 -> Switch3/2, Switch2/2
  Pdes/1 -> Switch2/1
  Switch2/1 -> Pbatt/1
  Constant1/1 -> Switch3/3
  Switch3/1 -> Qbatt/1
  Constant/1 -> Switch2/3
  Qdes/1 -> Switch3/1

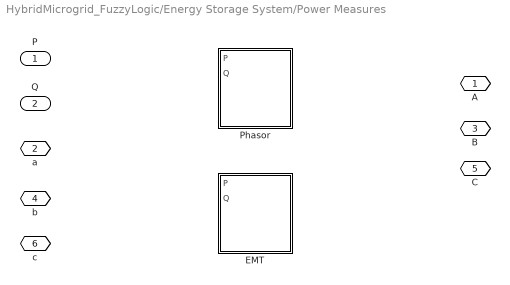
== system HybridMicrogrid_FuzzyLogic/Energy Storage System/Power Measures ==
  EMT : Subsystem  VariantControl=EMT
  Phasor : Subsystem  VariantControl=Phasor
  A : PMIOPort  Side=Left
  a : PMIOPort  Port=2  Side=Right
  B : PMIOPort  Port=3  Side=Left
  b : PMIOPort  Port=4  Side=Right
  C : PMIOPort  Port=5  Side=Left
  c : PMIOPort  Port=6  Side=Right
  P : Outport  VectorParamsAs1DForOutWhenUnconnected=off
  Q : Outport  Port=2  VectorParamsAs1DForOutWhenUnconnected=off

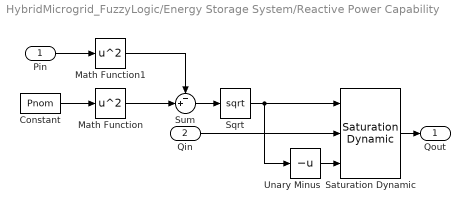
== system HybridMicrogrid_FuzzyLogic/Energy Storage System/Reactive Power Capability ==
  Pin : Inport
  Qin : Inport  Port=2
  Constant : Constant  Value=Pnom
  Math Function : Math  Operator=square  SignedPower=on
  Math Function1 : Math  Operator=square  SignedPower=on
  Saturation Dynamic : simulink/Discontinuities/Saturation Dynamic  OutMin=[]  OutMax=[]  OutDataTypeStr=Inherit: Same as second input  OutDataType=fixdt(1, 16)  OutScaling=2^-10  DoSatur=off
  Sqrt : Sqrt
  Sum : Sum  Inputs=-+|
  Unary Minus : UnaryMinus
  Qout : Outport  VectorParamsAs1DForOutWhenUnconnected=off
  wires:
  Sqrt/1 -> Saturation Dynamic/1, Unary Minus/1
  Math Function1/1 -> Sum/1
  Math Function/1 -> Sum/2
  Constant/1 -> Math Function/1
  Sum/1 -> Sqrt/1
  Unary Minus/1 -> Saturation Dynamic/3
  Saturation Dynamic/1 -> Qout/1
  Pin/1 -> Math Function1/1
  Qin/1 -> Saturation Dynamic/2

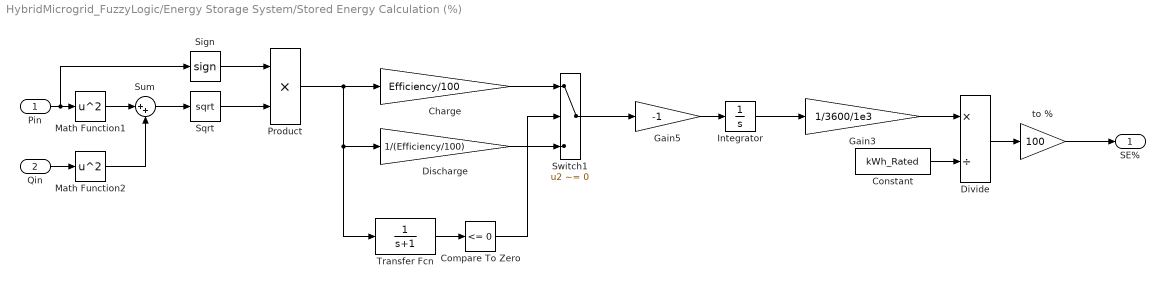
== system HybridMicrogrid_FuzzyLogic/Energy Storage System/Stored Energy Calculation (%) ==
  Pin : Inport
  Qin : Inport  Port=2
  Charge : Gain  Gain=Efficiency/100
  Compare To Zero : simulink/Logic and Bit Operations/Compare To Zero  relop=<=  OutDataTypeStr=boolean
  Constant : Constant  Value=kWh_Rated
  Discharge : Gain  Gain=1/(Efficiency/100)
  Divide : Product  Inputs=*/
  Gain3 : Gain  Gain=1/3600/1e3
  Gain5 : Gain  Gain=-1
  Integrator : Integrator  InitialCondition=(Initial_kWh_pc/100)*kWh_Rated*3600*1e3
  Math Function1 : Math  Operator=square  SignedPower=on
  Math Function2 : Math  Operator=square  SignedPower=on
  Product : Product
  Sign : Signum
  Sqrt : Sqrt
  Sum : Sum  Inputs=|++
  Switch1 : Switch  Criteria=u2 ~= 0  SaturateOnIntegerOverflow=off  InputSameDT=off
  Transfer Fcn : TransferFcn  Denominator=[1 1]
  to % : Gain  Gain=100
  SE% : Outport  VectorParamsAs1DForOutWhenUnconnected=off
  wires:
  Sign/1 -> Product/1
  Sqrt/1 -> Product/2
  Sum/1 -> Sqrt/1
  Math Function2/1 -> Sum/2
  Math Function1/1 -> Sum/1
  Qin/1 -> Math Function2/1
  Pin/1 -> Math Function1/1, Sign/1
  Product/1 -> Transfer Fcn/1, Discharge/1, Charge/1
  Discharge/1 -> Switch1/3
  Gain5/1 -> Integrator/1
  to %/1 -> SE%/1
  Transfer Fcn/1 -> Compare To Zero/1
  Switch1/1 -> Gain5/1
  Gain3/1 -> Divide/1
  Constant/1 -> Divide/2
  Charge/1 -> Switch1/1
  Divide/1 -> to %/1
  Compare To Zero/1 -> Switch1/2
  Integrator/1 -> Gain3/1

== system HybridMicrogrid_FuzzyLogic/Variable Load/Dynamic Load Control ==
  P0 : Inport
  Fcn : Fcn  Expr=sqrt(1/u(1)^2-1)
  Mux : Mux  Inputs=2
  Product : Product
  Summer1 : Constant  Value=PF
  PQ : Outport  VectorParamsAs1DForOutWhenUnconnected=off
  wires:
  Summer1/1 -> Fcn/1
  Fcn/1 -> Product/2
  P0/1 -> Product/1, Mux/1
  Mux/1 -> PQ/1
  Product/1 -> Mux/2  "Qo"

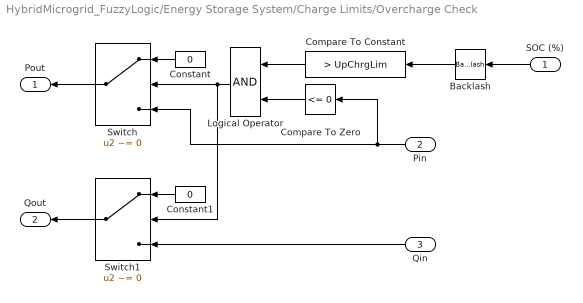
== system HybridMicrogrid_FuzzyLogic/Energy Storage System/Charge Limits/Overcharge Check ==
  SOC (%) : Inport
  Pin : Inport  Port=2
  Qin : Inport  Port=3
  Backlash : Backlash  BacklashWidth=1e-3  InitialOutput=Initial_kWh_pc  ZeroCross=off
  Compare To Constant : simulink/Logic and Bit Operations/Compare To Constant  relop=>  const=UpChrgLim  OutDataTypeStr=boolean
  Compare To Zero : simulink/Logic and Bit Operations/Compare To Zero  relop=<=  OutDataTypeStr=boolean
  Constant : Constant  Value=0
  Constant1 : Constant  Value=0
  Logical Operator : Logic  AllPortsSameDT=off  OutDataTypeStr=boolean
  Switch : Switch  Criteria=u2 ~= 0  SaturateOnIntegerOverflow=off  InputSameDT=off
  Switch1 : Switch  Criteria=u2 ~= 0  SaturateOnIntegerOverflow=off  InputSameDT=off
  Pout : Outport  VectorParamsAs1DForOutWhenUnconnected=off
  Qout : Outport  Port=2  VectorParamsAs1DForOutWhenUnconnected=off
  wires:
  Backlash/1 -> Compare To Constant/1
  Switch1/1 -> Qout/1
  Constant1/1 -> Switch1/1
  Qin/1 -> Switch1/3
  Compare To Zero/1 -> Logical Operator/2
  Switch/1 -> Pout/1
  Pin/1 -> Switch/3, Compare To Zero/1
  SOC (%)/1 -> Backlash/1
  Constant/1 -> Switch/1
  Logical Operator/1 -> Switch/2, Switch1/2
  Compare To Constant/1 -> Logical Operator/1

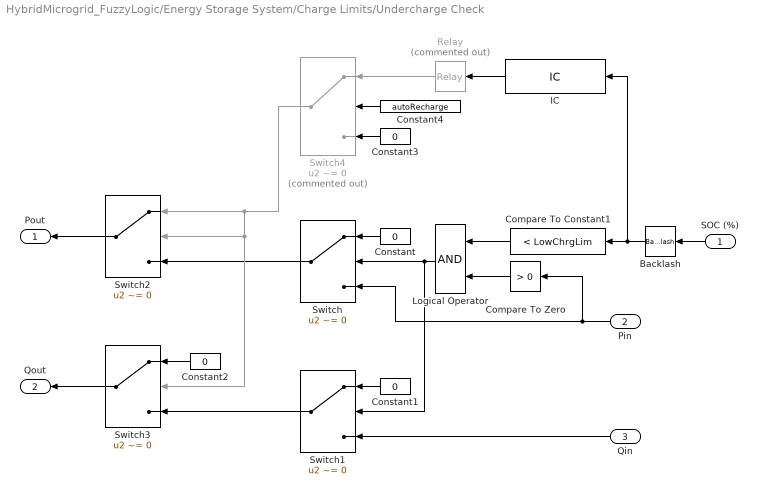
== system HybridMicrogrid_FuzzyLogic/Energy Storage System/Charge Limits/Undercharge Check ==
  SOC (%) : Inport
  Pin : Inport  Port=2
  Qin : Inport  Port=3
  Backlash : Backlash  BacklashWidth=1e-3  InitialOutput=Initial_kWh_pc  ZeroCross=off
  Compare To Constant1 : simulink/Logic and Bit Operations/Compare To Constant  relop=<  const=LowChrgLim  OutDataTypeStr=boolean
  Compare To Zero : simulink/Logic and Bit Operations/Compare To Zero  relop=>  OutDataTypeStr=boolean
  Constant{,1..3} (4 alike) : Constant  Value=0
  Constant4 : Constant  Value=autoRecharge
  IC : InitialCondition  Value=RechargeSOC
  Logical Operator : Logic  AllPortsSameDT=off  OutDataTypeStr=boolean
  Relay : Relay  Commented=on  OnSwitchValue=RechargeSOC  OffSwitchValue=LowChrgLim  OnOutputValue=0  OffOutputValue=-Precharge/100*Pnom
  Switch{,1..3} (4 alike) : Switch  Criteria=u2 ~= 0  SaturateOnIntegerOverflow=off  InputSameDT=off
  Switch4 : Switch  Commented=on  Criteria=u2 ~= 0  SaturateOnIntegerOverflow=off  InputSameDT=off
  Pout : Outport  VectorParamsAs1DForOutWhenUnconnected=off
  Qout : Outport  Port=2  VectorParamsAs1DForOutWhenUnconnected=off
  wires:
  Constant4/1 -> Switch4/2
  Constant3/1 -> Switch4/3
  Relay/1 -> Switch4/1
  Constant2/1 -> Switch3/1
  Switch1/1 -> Switch3/3
  Switch3/1 -> Qout/1
  Switch2/1 -> Pout/1
  Switch/1 -> Switch2/3
  IC/1 -> Relay/1
  Switch4/1 -> Switch3/2, Switch2/2, Switch2/1
  Backlash/1 -> Compare To Constant1/1, IC/1
  Qin/1 -> Switch1/3
  Constant1/1 -> Switch1/1
  Compare To Constant1/1 -> Logical Operator/1
  Logical Operator/1 -> Switch1/2, Switch/2
  Constant/1 -> Switch/1
  SOC (%)/1 -> Backlash/1
  Pin/1 -> Compare To Zero/1, Switch/3
  Compare To Zero/1 -> Logical Operator/2

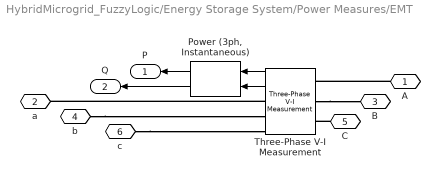
== system HybridMicrogrid_FuzzyLogic/Energy Storage System/Power Measures/EMT ==
  "Power (3ph, Instantaneous)" : powerlib_meascontrol/Measurements/Power (3ph, Instantaneous)
      settings: SourceProductName=Simscape Electrical
  Three-Phase V-I Measurement : powerlib/Measurements/Three-Phase V-I Measurement  VoltageMeasurement=phase-to-ground  SetLabelV=off  LabelV=Vabc  Vpu=off  VpuLL=off  CurrentMeasurement=yes  SetLabelI=off  LabelI=Iabc  Ipu=off  Pbase=100e6  Vbase=500e3  OutputType=Complex  PhasorSimulation=on  PSBequivalent=0
      settings: SourceProductName=Simscape Electrical
  A : PMIOPort  Side=Left
  a : PMIOPort  Port=2  Side=Right
  B : PMIOPort  Port=3  Side=Left
  b : PMIOPort  Port=4  Side=Right
  C : PMIOPort  Port=5  Side=Left
  c : PMIOPort  Port=6  Side=Right
  P : Outport  VectorParamsAs1DForOutWhenUnconnected=off
  Q : Outport  Port=2  VectorParamsAs1DForOutWhenUnconnected=off
  wires:
  Three-Phase V-I Measurement/2 -> "Power (3ph, Instantaneous)"/2
  Three-Phase V-I Measurement/1 -> "Power (3ph, Instantaneous)"/1
  "Power (3ph, Instantaneous)"/1 -> P/1
  "Power (3ph, Instantaneous)"/2 -> Q/1
  connections:
  Three-Phase V-I Measurement/RConn1 -- a/RConn1
  b/RConn1 -- Three-Phase V-I Measurement/RConn2
  A/RConn1 -- Three-Phase V-I Measurement/LConn1
  Three-Phase V-I Measurement/LConn2 -- B/RConn1
  c/RConn1 -- Three-Phase V-I Measurement/RConn3
  C/RConn1 -- Three-Phase V-I Measurement/LConn3

== system HybridMicrogrid_FuzzyLogic/Energy Storage System/Power Measures/Phasor ==
  "Power (3ph, Phasor)" : spsPower3phPhasorLib/Power (3ph, Phasor)
      settings: LibrarySourceBlock=|
      | sps_lib/Sensors and Measurements/Power
      | (3ph, Phasor)
  Three-Phase V-I Measurement : spsThreePhaseVIMeasurementLib/Three-Phase V-I Measurement  VoltageMeasurement=phase-to-ground  SetLabelV=off  LabelV=Vabc  Vpu=off  VpuLL=off  CurrentMeasurement=yes  SetLabelI=off  LabelI=Iabc  Ipu=off  Pbase=100e6  Vbase=500e3  OutputType=Complex  PhasorSimulation=on  PSBequivalent=0
  A : PMIOPort  Side=Left
  a : PMIOPort  Port=2  Side=Right
  B : PMIOPort  Port=3  Side=Left
  b : PMIOPort  Port=4  Side=Right
  C : PMIOPort  Port=5  Side=Left
  c : PMIOPort  Port=6  Side=Right
  P : Outport  VectorParamsAs1DForOutWhenUnconnected=off
  Q : Outport  Port=2  VectorParamsAs1DForOutWhenUnconnected=off
  wires:
  "Power (3ph, Phasor)"/2 -> Q/1
  "Power (3ph, Phasor)"/1 -> P/1
  Three-Phase V-I Measurement/1 -> "Power (3ph, Phasor)"/1
  Three-Phase V-I Measurement/2 -> "Power (3ph, Phasor)"/2
  connections:
  C/RConn1 -- Three-Phase V-I Measurement/LConn3
  c/RConn1 -- Three-Phase V-I Measurement/RConn3
  Three-Phase V-I Measurement/LConn2 -- B/RConn1
  A/RConn1 -- Three-Phase V-I Measurement/LConn1
  b/RConn1 -- Three-Phase V-I Measurement/RConn2
  Three-Phase V-I Measurement/RConn1 -- a/RConn1

== matlab function HybridMicrogrid_FuzzyLogic/MATLAB Function3 ==
  settings: updateMethod=DISCRETE
  data: time input; total_cost output; price input; power input
function total_cost = calculateGridEnergyCost(time, price, power)
% Inputs:
%   time - Current simulation time (s)
%   price - Current electricity price ($/kWh)
%   power - Current grid import power (kW) (positive = importing)

% Output:
%   total_cost - Running total of energy costs ($)

persistent cumulative_cost;
persistent last_time;

% Initialize
if isempty(cumulative_cost)
    cumulative_cost = 0;
    last_time = 0;
end

% Calculate time step in hours
dt = (time - last_time)/3600;

% Only calculate if time has advanced
if dt > 0
    % Cost = power (kW) * time (h) * price (R/kWh)
    % Only count positive power (importing)
    if power > 0
        cumulative_cost = cumulative_cost + power * dt * price;
    end
end

% Update time for next step
last_time = time;

% Output the total
total_cost = cumulative_cost;
end
